simulink model "model_2_klatna_i_opruge"  (R2015a)
settings: Solver=ode45  StartTime=0.0  StopTime=300  RelTol=1e-3
values from neighbouring files (symbols this model uses):
  teta1 = 0.5    [Parametri.m]
  teta2 = -0    (= 0)    [Parametri.m]
  v1 = 0    [Parametri.m]
  v2 = 0    [Parametri.m]
settings Model: Creator=BLAGI  LastModifiedBy=BLAGI

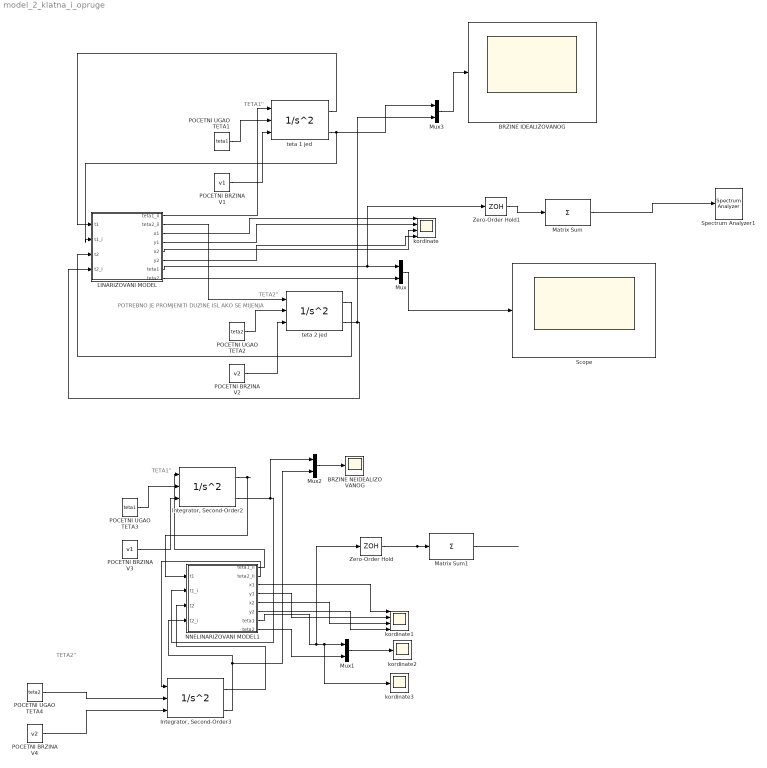
== system model_2_klatna_i_opruge ==
  note: POTREBNO JE PROMJENITI DUZINE ISL AKO
      | SE MIJENJA
  note: TETA1''
  note: TETA2''
  note: TETA1''
  note: TETA2''
  BRZINE IDEALIZOVANOG : Scope
      settings: ShowLegends=on  SaveName=ScopeData7
  BRZINE NEIDEALIZOVANOG : Scope
      settings: ShowLegends=on  SaveName=ScopeData6
  "Integrator, Second-Order2" : SecondOrderIntegrator  ICSourceX=external  LimitX=on  UpperLimitX=45  LowerLimitX=-45  ICSourceDXDT=external  LimitDXDT=on  UpperLimitDXDT=200  LowerLimitDXDT=-200
  "Integrator, Second-Order3" : SecondOrderIntegrator  ICSourceX=external  LimitX=on  UpperLimitX=45  LowerLimitX=-45  ICSourceDXDT=external  LimitDXDT=on  UpperLimitDXDT=200  LowerLimitDXDT=-200
  LINARIZOVANI MODEL : MATLAB Function  TreatAsAtomicUnit=on
  Matrix Sum : Sum  Inputs=+
  Matrix Sum1 : Sum  Inputs=+
  Mux{,1..3} (4 alike) : Mux  Inputs=2
  NNELINARIZOVANI MODEL1 : MATLAB Function  TreatAsAtomicUnit=on
  POCETNI BRZINA V1 : Constant  Value=v1
  POCETNI BRZINA V2 : Constant  Value=v2
  POCETNI BRZINA V3 : Constant  Value=v1
  POCETNI BRZINA V4 : Constant  Value=v2
  POCETNI UGAO TETA1 : Constant  Value=teta1
  POCETNI UGAO TETA2 : Constant  Value=teta2
  POCETNI UGAO TETA3 : Constant  Value=teta1
  POCETNI UGAO TETA4 : Constant  Value=teta2
  Scope : Scope
      settings: SaveName=ScopeData2
  Spectrum Analyzer1 : SpectrumAnalyzer
  Zero-Order Hold : ZeroOrderHold  SampleTime=0.01
  Zero-Order Hold1 : ZeroOrderHold  SampleTime=0.01
  kordinate : Scope  NumInputPorts=4
      settings: ShowLegends=on  YMin=-5~-5~-5~-5  YMax=5~5~5~5
  kordinate1 : Scope  NumInputPorts=4
      settings: ShowLegends=on  YMin=-5~-5~-5~-5  YMax=5~5~5~5  SaveName=ScopeData3
  kordinate2 : Scope
      settings: ShowLegends=on  SaveName=ScopeData4
  kordinate3 : Scope
      settings: ShowLegends=on  SaveName=ScopeData5
  teta 1 jed : SecondOrderIntegrator  ICSourceX=external  ICSourceDXDT=external
  teta 2 jed : SecondOrderIntegrator  ICSourceX=external  ICSourceDXDT=external
  wires:
  LINARIZOVANI MODEL/1(teta1_ii) -> teta 1 jed/1
  POCETNI UGAO TETA1/1 -> teta 1 jed/2
  POCETNI BRZINA V1/1 -> teta 1 jed/3
  POCETNI UGAO TETA2/1 -> teta 2 jed/2
  POCETNI BRZINA V2/1 -> teta 2 jed/3
  LINARIZOVANI MODEL/2(teta2_ii) -> teta 2 jed/1
  teta 1 jed/1 -> LINARIZOVANI MODEL/1(t1)
  teta 1 jed/2 -> Mux3/1, LINARIZOVANI MODEL/2(t1_i)
  teta 2 jed/1 -> LINARIZOVANI MODEL/3(t2)
  teta 2 jed/2 -> Mux3/2, LINARIZOVANI MODEL/4(t2_i)
  LINARIZOVANI MODEL/3(x1) -> kordinate/1
  LINARIZOVANI MODEL/4(y1) -> kordinate/2
  LINARIZOVANI MODEL/5(x2) -> kordinate/3
  LINARIZOVANI MODEL/6(y2) -> kordinate/4
  Mux/1 -> Scope/1
  LINARIZOVANI MODEL/7(teta1) -> Zero-Order Hold1/1, Mux/1
  LINARIZOVANI MODEL/8(teta2) -> Mux/2
  POCETNI UGAO TETA3/1 -> "Integrator, Second-Order2"/2
  POCETNI BRZINA V3/1 -> "Integrator, Second-Order2"/3
  POCETNI UGAO TETA4/1 -> "Integrator, Second-Order3"/2
  POCETNI BRZINA V4/1 -> "Integrator, Second-Order3"/3
  NNELINARIZOVANI MODEL1/1(teta1_ii) -> "Integrator, Second-Order2"/1
  NNELINARIZOVANI MODEL1/2(teta2_ii) -> "Integrator, Second-Order3"/1
  NNELINARIZOVANI MODEL1/3(x1) -> kordinate1/1
  NNELINARIZOVANI MODEL1/4(y1) -> kordinate1/2
  NNELINARIZOVANI MODEL1/5(x2) -> kordinate1/3
  NNELINARIZOVANI MODEL1/6(y2) -> kordinate1/4
  Mux1/1 -> kordinate2/1
  "Integrator, Second-Order2"/1 -> NNELINARIZOVANI MODEL1/1(t1)
  "Integrator, Second-Order3"/1 -> NNELINARIZOVANI MODEL1/3(t2)
  "Integrator, Second-Order2"/2 -> Mux2/1, NNELINARIZOVANI MODEL1/2(t1_i)
  "Integrator, Second-Order3"/2 -> Mux2/2, NNELINARIZOVANI MODEL1/4(t2_i)
  NNELINARIZOVANI MODEL1/7(teta1) -> Zero-Order Hold/1, kordinate3/1, Mux1/1
  NNELINARIZOVANI MODEL1/8(teta2) -> Mux1/2
  Mux2/1 -> BRZINE NEIDEALIZOVANOG/1
  Zero-Order Hold1/1 -> Matrix Sum/1
  Mux3/1 -> BRZINE IDEALIZOVANOG/1
  Zero-Order Hold/1 -> Matrix Sum1/1
  Matrix Sum1/1 -> ?
  Matrix Sum/1 -> Spectrum Analyzer1/1

== matlab function model_2_klatna_i_opruge/NNELINARIZOVANI MODEL1 ==
  data: t1 input; teta1_ii output; t1_i input; t2 input; teta2_ii output; t2_i input; x1 output; y1 output; x2 output; y2 output; teta1 output; teta2 output
function [teta1_ii,teta2_ii,x1,y1,x2,y2,teta1,teta2] = fcn(t1,t1_i,t2,t2_i)
%#codegen  
m1=1;
m2=1;
k=1;
l1=5;
l2=5;
g=9.81;
teta1_ii =1/l1/m1/cos(t1)*((m1*g*tan(t1)+k*l1*sin(t1)-k*l2*sin(t2)-l1*m1*t1_i*t1_i*sin(t1))); 
teta2_ii =1/l2/m2/cos(t2)*((m2*g*tan(t2)+k*l2*sin(t2)-k*l1*sin(t1)-l2*m2*t2_i*t2_i*sin(t2))); 
x1=l1*sin(t1);
y1=-l1*sin(t1);
x2=l2*sin(t2);
y2=l2*sin(t2);
teta1=t1;
teta2=t2;

== matlab function model_2_klatna_i_opruge/LINARIZOVANI MODEL ==
  data: t1 input; teta1_ii output; t1_i input; t2 input; teta2_ii output; t2_i input; x1 output; y1 output; x2 output; y2 output; teta1 output; teta2 output
function [teta1_ii,teta2_ii,x1,y1,x2,y2,teta1,teta2] = fcn(t1,t1_i,t2,t2_i)
%#codegen  
m1=1;
m2=1;
k=1;
l1=5;
l2=5;
g=9.81;
teta1_ii = -1/l1/m1/cos(t1)*((m1*g+k*l1-l1*m1*t1_i*t1_i)*sin(t1)-k*l2*sin(t2));
teta2_ii=-1/l2/m2/cos(t2)*((m2*g+k*l2-l2*m2*t2_i*t2_i)*sin(t2)-k*l2*sin(t1));
x1=l1*sin(t1);
y1=-l1*sin(t1);
x2=l2*sin(t2);
y2=l2*sin(t2);
teta1=t1;
teta2=t2;
